simulink model "Full_system_6DOF"  (R2015b)
settings: Solver=ode3  StartTime=0.0  StopTime=30  FixedStep=0.001  RelTol=1e-3
values from neighbouring files (symbols this model uses):
  CoM = [0,0.00934172358962716,0.00356822089773090]'    [init_sim_3DOF.m]    (also in init_sim_4DOF.m = [0,0,0]'; init_sim_6DOF.m = [0,-0.01,0]')
  OS_damping_rot = 0    [init_sim_4DOF.m]    (also in init_sim_6DOF.m)
  OS_damping_trans = 0    [init_sim_4DOF.m]    (also in init_sim_6DOF.m)
  OS_Inertia = 1e-9*[13894080.33 -19869.26 46055.05 ... (first row only)    [init_sim_1DOF.m]    (also in init_sim_3DOF.m; init_sim_4DOF.m; init_sim_6DOF.m = 1e-9*[15414004.18 -17587.97 46447.37)
  OS_init_omega = 0    [init_sim_1DOF.m]    (also in init_sim_3DOF.m; init_sim_4DOF.m = [0 0 0]'; init_sim_6DOF.m = [0 0 0]')
  OS_init_vel = [0,0,0]'    [init_sim_3DOF.m]    (also in init_sim_4DOF.m; init_sim_6DOF.m)
  OS_rotation = 0    [init_sim_1DOF.m]    (also in init_sim_3DOF.m; init_sim_4DOF.m = [0 0 0]'; init_sim_6DOF.m = [0 0 0]')
  OS_xyz_des = (ea2dcm(SC_xyz(1,:)',72*pi/180)*OS_xyz_0')'    [init_sim_3DOF.m]    (also in init_sim_4DOF.m; init_sim_6DOF.m)
  rot_gain = 1e-8    (= 1e-08)    [init_sim_3DOF.m]    (also in init_sim_4DOF.m; init_sim_6DOF.m)
  SROA_Inertia = 1e7*eye(3)    [init_sim_3DOF.m]    (also in init_sim_4DOF.m)
  SROA_Mass = 100000    [init_sim_3DOF.m]    (also in init_sim_4DOF.m)
  trans_gain = 1e-7    (= 1e-07)    [init_sim_3DOF.m]    (also in init_sim_4DOF.m; init_sim_6DOF.m)
undefined symbols (not defined in the file or in its folder): EM_mu, EM_xyz, origin, OS_Mass, OS_mu_0, OS_xyz_0, Quat_A0
libraries: vrlib x3, simulink x3, my_ACS_library x1
settings Model: Creator=Frances  LastModifiedBy=user
settings DataIOCC: SaveFormat=Array
settings DebuggingCC: MaxConsecutiveZCsMsg=none  SolverPrmCheckMsg=warning
settings HardwareCC: ProdBitPerPointer=32  ProdLargestAtomicFloat=None  ProdIntDivRoundTo=Undefined  ProdEndianess=Unspecified  ProdWordSize=32  ProdHWDeviceType=32-bit Generic
settings GRTTargetCC: GeneratePreprocessorConditionals=Disable all
settings ConfigComp: CovModelRefEnable=Off  CovSFcnEnable=off

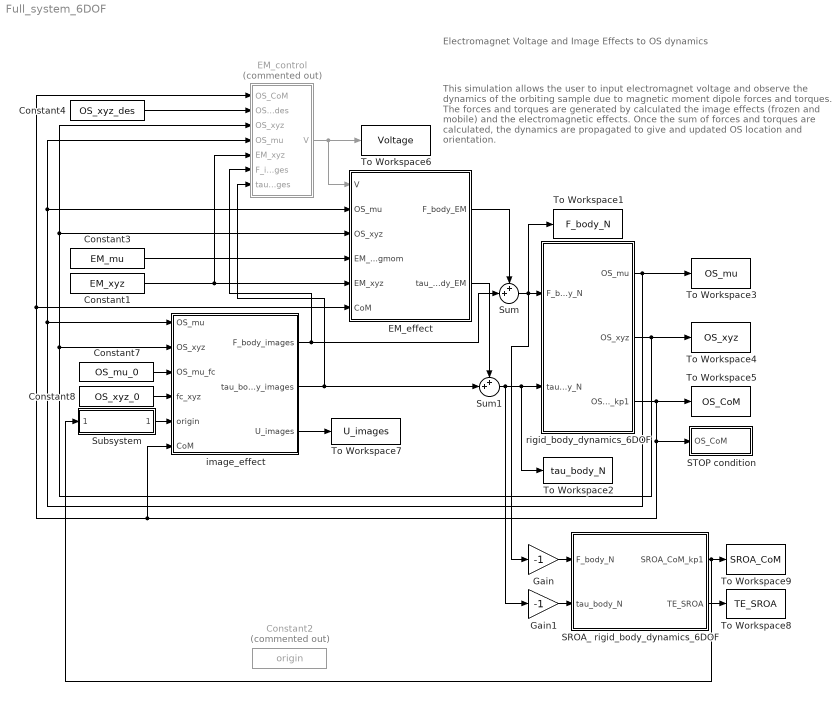
== system Full_system_6DOF ==
  note: This simulation allows the user to input electromagnet voltage and observe
      | the dynamics of the orbiting sample due to magnetic moment dipole forces
      | and torques. The forces and torques are generated by calculated the image
      | effects (frozen and mobile) and the electromagnetic effects. Once the sum
      | of forces and torques are calculated, the dynamics are propagated to give
      | and updated OS location and orientation.
  note: Electromagnet Voltage and Image Effects
      | to OS dynamics
  Constant1 : Constant  Value=EM_xyz
  Constant2 : Constant  Commented=on  Value=origin
  Constant3 : Constant  Value=EM_mu
  Constant4 : Constant  Value=OS_xyz_des
  Constant7 : Constant  Value=OS_mu_0  VectorParams1D=off
  Constant8 : Constant  Value=OS_xyz_0
  EM_control : Subsystem  Commented=on
  EM_effect : MATLAB Function  TreatAsAtomicUnit=on
  Gain : Gain  Gain=-1
  Gain1 : Gain  Gain=-1
  SROA_ rigid_body_dynamics_6DOF : Subsystem
  STOP condition : Subsystem
  Subsystem : Subsystem
  Sum : Sum  Inputs=++|
  Sum1 : Sum  Inputs=++|
  To Workspace1 : ToWorkspace  VariableName=F_body_N  SaveFormat=Timeseries  SampleTime=-1
  To Workspace2 : ToWorkspace  VariableName=tau_body_N  SaveFormat=Timeseries  SampleTime=-1
  To Workspace3 : ToWorkspace  VariableName=OS_mu  SaveFormat=Timeseries  SampleTime=-1
  To Workspace4 : ToWorkspace  VariableName=OS_xyz  SaveFormat=Timeseries  SampleTime=-1
  To Workspace5 : ToWorkspace  VariableName=OS_CoM  SaveFormat=Timeseries  SampleTime=-1
  To Workspace6 : ToWorkspace  VariableName=Voltage  SaveFormat=Timeseries  SampleTime=-1
  To Workspace7 : ToWorkspace  VariableName=U_images  SaveFormat=Timeseries  SampleTime=-1
      settings: Save2DSignal=2-D array (concatenate along first dimension)
  To Workspace8 : ToWorkspace  VariableName=TE_SROA  SaveFormat=Timeseries  SampleTime=-1
  To Workspace9 : ToWorkspace  VariableName=SROA_CoM  SaveFormat=Timeseries  SampleTime=-1
  image_effect : MATLAB Function  TreatAsAtomicUnit=on
  "rigid_body_dynamics_6DOF " : Subsystem
  wires:
  Constant3/1 -> EM_effect/4(EM_magmom)
  Constant1/1 -> EM_effect/5(EM_xyz), EM_control/5(EM_xyz)
  Subsystem/1(SROA_origin) -> image_effect/5(origin)
  Constant7/1 -> image_effect/3(OS_mu_fc)
  Constant8/1 -> image_effect/4(fc_xyz)
  image_effect/1(F_body_images) -> EM_control/6(F_images), Sum/2
  EM_effect/1(F_body_EM) -> Sum/1
  image_effect/2(tau_body_images) -> Sum1/2, EM_control/7(tau_images)
  EM_effect/2(tau_body_EM) -> Sum1/1
  Sum/1 -> To Workspace1/1, Gain/1, "rigid_body_dynamics_6DOF "/1(F_body_N)
  Sum1/1 -> Gain1/1, To Workspace2/1, "rigid_body_dynamics_6DOF "/2(tau_body_N)
  "rigid_body_dynamics_6DOF "/1(OS_mu) -> To Workspace3/1, EM_control/4(OS_mu), EM_effect/2(OS_mu), image_effect/1(OS_mu)
  "rigid_body_dynamics_6DOF "/2(OS_xyz) -> To Workspace4/1, EM_effect/3(OS_xyz), EM_control/3(OS_xyz), image_effect/2(OS_xyz)
  image_effect/3(U_images) -> To Workspace7/1
  "rigid_body_dynamics_6DOF "/3(OS_CoM_kp1) -> image_effect/6(CoM), EM_control/1(OS_CoM), EM_effect/6(CoM), STOP condition/1(OS_CoM), To Workspace5/1
  EM_control/1(V) -> EM_effect/1(V), To Workspace6/1
  Constant4/1 -> EM_control/2(OS_xyz_des)
  Gain/1 -> SROA_ rigid_body_dynamics_6DOF/1(F_body_N)
  Gain1/1 -> SROA_ rigid_body_dynamics_6DOF/2(tau_body_N)
  SROA_ rigid_body_dynamics_6DOF/2(TE_SROA) -> To Workspace8/1
  SROA_ rigid_body_dynamics_6DOF/1(SROA_CoM_kp1) -> Subsystem/1(SROA_CoM), To Workspace9/1

== system Full_system_6DOF/EM_control ==
  OS_CoM : Inport
  OS_xyz_des : Inport  Port=2
  OS_xyz : Inport  Port=3
  OS_mu : Inport  Port=4
  EM_xyz : Inport  Port=5
  F_images : Inport  Port=6
  tau_images : Inport  Port=7
  Display : Display
  calculate_V : Subsystem
  desired : Subsystem
  V : Outport
  wires:
  OS_xyz/1 -> desired/3(OS_xyz)
  OS_mu/1 -> desired/4(OS_mu)
  EM_xyz/1 -> desired/5(EM_xyz)
  OS_xyz_des/1 -> desired/2(OS_xyz_des)
  OS_CoM/1 -> desired/1(OS_CoM)
  calculate_V/1(V) -> Display/1, V/1
  F_images/1 -> desired/6(F_images)
  tau_images/1 -> desired/7(tau_images)
  desired/1(F_des) -> calculate_V/1(F_em)
  desired/2(tau_des) -> calculate_V/2(tau_em)
  desired/3(d/dV) -> calculate_V/3(dV)

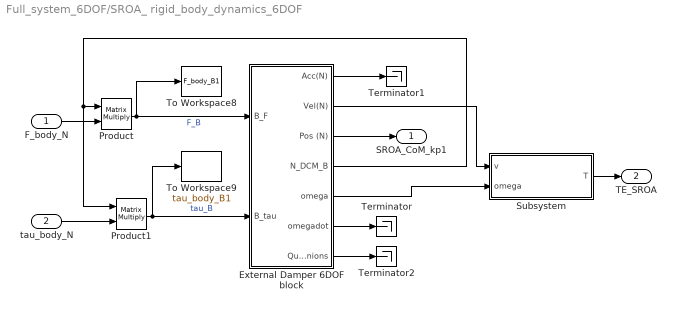
== system Full_system_6DOF/SROA_ rigid_body_dynamics_6DOF ==
  F_body_N : Inport
  tau_body_N : Inport  Port=2
  External Damper 6DOF block : Subsystem
  Product : Product  Multiplication=Matrix(*)
  Product1 : Product  Multiplication=Matrix(*)
  Subsystem : Subsystem
  Terminator : Terminator
  Terminator1 : Terminator
  Terminator2 : Terminator
  To Workspace8 : ToWorkspace  VariableName=F_body_B1  SaveFormat=Timeseries  SampleTime=-1
  To Workspace9 : ToWorkspace  VariableName=tau_body_B1  SaveFormat=Timeseries  SampleTime=-1
  SROA_CoM_kp1 : Outport
  TE_SROA : Outport  Port=2  PortDimensions=1
  wires:
  External Damper 6DOF block/1(Acc(N)) -> Terminator1/1
  External Damper 6DOF block/6(omegadot) -> Terminator/1
  tau_body_N/1 -> Product1/2
  F_body_N/1 -> Product/2
  External Damper 6DOF block/4(N_DCM_B) -> Product1/1, Product/1
  Product1/1 -> External Damper 6DOF block/2(B_tau), To Workspace9/1  "tau_B"
  Product/1 -> To Workspace8/1, External Damper 6DOF block/1(B_F)  "F_B"
  External Damper 6DOF block/3(Pos (N)) -> SROA_CoM_kp1/1
  Subsystem/1(T) -> TE_SROA/1
  External Damper 6DOF block/2(Vel(N)) -> Subsystem/1(v)
  External Damper 6DOF block/5(omega) -> Subsystem/2(omega)
  External Damper 6DOF block/7(Quaternions) -> Terminator2/1

== system Full_system_6DOF/STOP condition ==
  OS_CoM : Inport
  Compare To Constant : simulink/Logic and Bit Operations/Compare To Constant  relop=>  const=0.1  OutDataTypeStr=boolean
  Stop Simulation : Stop
  norm : Fcn  Expr=sqrt(u(1)^2+u(2)^2+u(3)^2)
  wires:
  Compare To Constant/1 -> Stop Simulation/1
  norm/1 -> Compare To Constant/1
  OS_CoM/1 -> norm/1

== system Full_system_6DOF/Subsystem ==
  SROA_CoM : Inport
  Constant2 : Constant  Value=origin
  MATLAB Function : MATLAB Function  TreatAsAtomicUnit=on
  SROA_origin : Outport
  wires:
  Constant2/1 -> MATLAB Function/1(origin)
  SROA_CoM/1 -> MATLAB Function/2(CoM)
  MATLAB Function/1(origin_new) -> SROA_origin/1

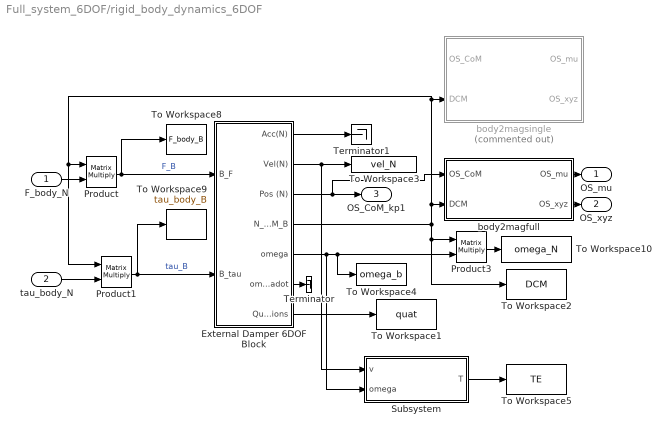
== system Full_system_6DOF/rigid_body_dynamics_6DOF  ==
  F_body_N : Inport
  tau_body_N : Inport  Port=2
  External Damper 6DOF Block : Subsystem
  Product : Product  Multiplication=Matrix(*)
  Product1 : Product  Multiplication=Matrix(*)
  Product3 : Product  Multiplication=Matrix(*)
  Subsystem : Subsystem
  Terminator : Terminator
  Terminator1 : Terminator
  To Workspace1 : ToWorkspace  VariableName=quat  SaveFormat=Timeseries  SampleTime=-1
  To Workspace10 : ToWorkspace  VariableName=omega_N  SaveFormat=Timeseries  SampleTime=-1
  To Workspace2 : ToWorkspace  VariableName=DCM  SaveFormat=Structure With Time  SampleTime=-1
  To Workspace3 : ToWorkspace  VariableName=vel_N  SaveFormat=Timeseries  SampleTime=-1
  To Workspace4 : ToWorkspace  VariableName=omega_b  SaveFormat=Timeseries  SampleTime=-1
  To Workspace5 : ToWorkspace  VariableName=TE  SaveFormat=Timeseries  SampleTime=-1
  To Workspace8 : ToWorkspace  VariableName=F_body_B  SaveFormat=Timeseries  SampleTime=-1
  To Workspace9 : ToWorkspace  VariableName=tau_body_B  SaveFormat=Timeseries  SampleTime=-1
  body2magfull : MATLAB Function  TreatAsAtomicUnit=on
  body2magsingle : MATLAB Function  Commented=on  TreatAsAtomicUnit=on
  OS_mu : Outport
  OS_xyz : Outport  Port=2
  OS_CoM_kp1 : Outport  Port=3
  wires:
  External Damper 6DOF Block/1(Acc(N)) -> Terminator1/1
  External Damper 6DOF Block/6(omegadot) -> Terminator/1
  External Damper 6DOF Block/2(Vel(N)) -> Subsystem/1(v), To Workspace3/1
  body2magfull/2(OS_xyz) -> OS_xyz/1
  body2magfull/1(OS_mu) -> OS_mu/1
  tau_body_N/1 -> Product1/2
  F_body_N/1 -> Product/2
  External Damper 6DOF Block/4(N_DCM_B) -> body2magfull/2(DCM), body2magsingle/2(DCM), Product1/1, Product/1, Product3/1, To Workspace2/1
  Product1/1 -> External Damper 6DOF Block/2(B_tau), To Workspace9/1  "tau_B"
  Product/1 -> External Damper 6DOF Block/1(B_F), To Workspace8/1  "F_B"
  External Damper 6DOF Block/3(Pos (N)) -> OS_CoM_kp1/1, body2magfull/1(OS_CoM)
  Product3/1 -> To Workspace10/1
  External Damper 6DOF Block/5(omega) -> Product3/2, To Workspace4/1, Subsystem/2(omega)
  External Damper 6DOF Block/7(Quaternions) -> To Workspace1/1
  Subsystem/1(T) -> To Workspace5/1

== system Full_system_6DOF/EM_control/calculate_V ==
  F_em : Inport
  tau_em : Inport  Port=2
  dV : Inport  Port=3
  Abs : Abs
  Divide : Product  Inputs=*/
  Gain : Gain  Gain=12
  MATLAB Function : MATLAB Function  TreatAsAtomicUnit=on
  MinMax : MinMax  Function=max
  Saturation : Saturate  Commented=on  UpperLimit=12  LowerLimit=-12  ZeroCross=off
  V : Outport
  wires:
  dV/1 -> MATLAB Function/3(dV)
  tau_em/1 -> MATLAB Function/2(tau_em)
  F_em/1 -> MATLAB Function/1(F_em)
  MinMax/1 -> Divide/2
  Abs/1 -> MinMax/1
  Divide/1 -> Gain/1
  MATLAB Function/1(V) -> Abs/1, Divide/1
  Gain/1 -> V/1

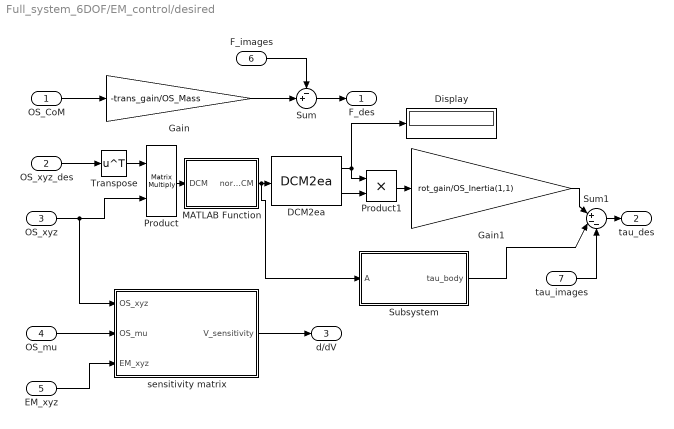
== system Full_system_6DOF/EM_control/desired ==
  OS_CoM : Inport
  OS_xyz_des : Inport  Port=2
  OS_xyz : Inport  Port=3
  OS_mu : Inport  Port=4
  EM_xyz : Inport  Port=5
  F_images : Inport  Port=6
  tau_images : Inport  Port=7
  DCM2ea : my_ACS_library/attitude conversions/DCM2ea
  Display : Display
  Gain : Gain  Gain=-trans_gain/OS_Mass
  Gain1 : Gain  Gain=rot_gain/OS_Inertia(1,1)
  MATLAB Function : MATLAB Function  TreatAsAtomicUnit=on
  Product : Product  Multiplication=Matrix(*)
  Product1 : Product
  Subsystem : Subsystem
  Sum : Sum  Inputs=-+|
  Sum1 : Sum  Inputs=|+--
  Transpose : Math  Operator=transpose  SaturateOnIntegerOverflow=on
  sensitivity matrix : MATLAB Function  TreatAsAtomicUnit=on
  F_des : Outport
  tau_des : Outport  Port=2
  d/dV : Outport  Port=3
  wires:
  sensitivity matrix/1(V_sensitivity) -> d/dV/1
  OS_xyz_des/1 -> Transpose/1
  Transpose/1 -> Product/1
  OS_CoM/1 -> Gain/1
  EM_xyz/1 -> sensitivity matrix/3(EM_xyz)
  OS_xyz/1 -> Product/2, sensitivity matrix/1(OS_xyz)
  OS_mu/1 -> sensitivity matrix/2(OS_mu)
  Product/1 -> MATLAB Function/1(DCM)
  MATLAB Function/1(normDCM) -> Subsystem/1(A), DCM2ea/1
  Product1/1 -> Gain1/1
  DCM2ea/1 -> Product1/1, Display/1
  DCM2ea/2 -> Product1/2
  Gain/1 -> Sum/2
  Sum/1 -> F_des/1
  F_images/1 -> Sum/1
  Sum1/1 -> tau_des/1
  Gain1/1 -> Sum1/1
  tau_images/1 -> Sum1/3
  Subsystem/1(tau_body) -> Sum1/2

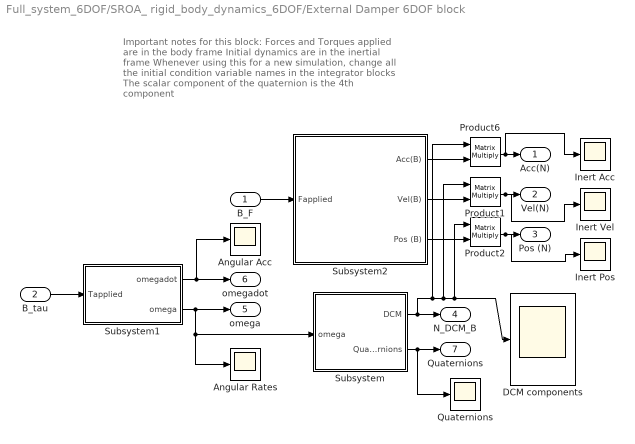
== system Full_system_6DOF/SROA_ rigid_body_dynamics_6DOF/External Damper 6DOF block ==
  note: Important notes for this block:
      | Forces and Torques applied are in the body frame
      | Initial dynamics are in the inertial frame
      | Whenever using this for a new simulation, change all the initial condition variable names in the integrator blocks
      | The scalar component of the quaternion is the 4th component
  B_F : Inport
  B_tau : Inport  Port=2
  Angular Acc : Scope
  Angular Rates : Scope
  DCM components : Scope
  Inert Acc : Scope
  Inert Pos : Scope
  Inert Vel : Scope
  Product1 : Product  Multiplication=Matrix(*)  RndMeth=Zero
  Product2 : Product  Multiplication=Matrix(*)  RndMeth=Zero
  Product6 : Product  Multiplication=Matrix(*)  RndMeth=Zero
  "Quaternions " : Scope
  Subsystem : Subsystem
  Subsystem1 : Subsystem
  Subsystem2 : Subsystem
  Acc(N) : Outport
  Vel(N) : Outport  Port=2
  Pos (N) : Outport  Port=3
  N_DCM_B : Outport  Port=4
  omega : Outport  Port=5
  omegadot : Outport  Port=6
  Quaternions : Outport  Port=7
  wires:
  Subsystem/2(Quaternions) -> Quaternions/1, "Quaternions "/1
  Subsystem/1(DCM) -> N_DCM_B/1, Product6/1, Product1/1, Product2/1, DCM components/1
  Subsystem1/1(omegadot) -> omegadot/1, Angular Acc/1
  Subsystem1/2(omega) -> Angular Rates/1, Subsystem/1(omega), omega/1
  B_F/1 -> Subsystem2/1(Fapplied)
  B_tau/1 -> Subsystem1/1(Tapplied)
  Product6/1 -> Inert Acc/1, Acc(N)/1
  Product1/1 -> Inert Vel/1, Vel(N)/1
  Product2/1 -> Inert Pos/1, Pos (N)/1
  Subsystem2/2(Vel(B)) -> Product1/2
  Subsystem2/1(Acc(B)) -> Product6/2
  Subsystem2/3(Pos (B)) -> Product2/2

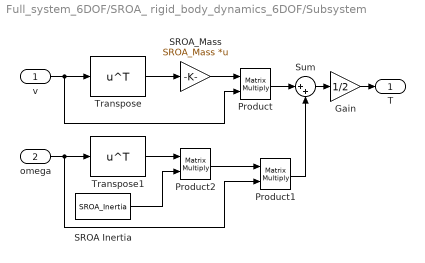
== system Full_system_6DOF/SROA_ rigid_body_dynamics_6DOF/Subsystem ==
  v : Inport
  omega : Inport  Port=2
  Gain : Gain  Gain=1/2
  Product : Product  Multiplication=Matrix(*)
  Product1 : Product  Multiplication=Matrix(*)
  Product2 : Product  Multiplication=Matrix(*)
  SROA Inertia : Constant  Value=SROA_Inertia
  SROA_Mass : Gain  Gain=SROA_Mass  Multiplication=Matrix(K*u)
  Sum : Sum  Inputs=|++
  Transpose : Math  Operator=transpose  SaturateOnIntegerOverflow=on
  Transpose1 : Math  Operator=transpose  SaturateOnIntegerOverflow=on
  T : Outport
  wires:
  v/1 -> Product/2, Transpose/1
  Transpose/1 -> SROA_Mass/1
  SROA_Mass/1 -> Product/1
  Sum/1 -> Gain/1
  Gain/1 -> T/1
  omega/1 -> Product1/2, Transpose1/1
  Transpose1/1 -> Product2/1
  Product2/1 -> Product1/1
  Product/1 -> Sum/1
  Product1/1 -> Sum/2
  SROA Inertia/1 -> Product2/2

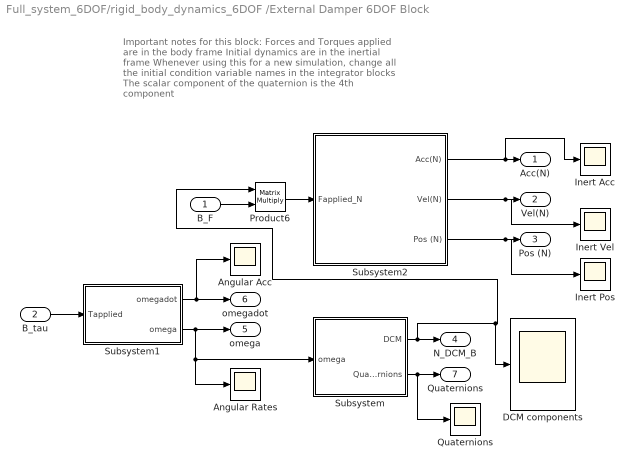
== system Full_system_6DOF/rigid_body_dynamics_6DOF /External Damper 6DOF Block ==
  note: Important notes for this block:
      | Forces and Torques applied are in the body frame
      | Initial dynamics are in the inertial frame
      | Whenever using this for a new simulation, change all the initial condition variable names in the integrator blocks
      | The scalar component of the quaternion is the 4th component
  B_F : Inport
  B_tau : Inport  Port=2
  Angular Acc : Scope
  Angular Rates : Scope
  DCM components : Scope
  Inert Acc : Scope
  Inert Pos : Scope
  Inert Vel : Scope
  Product6 : Product  Multiplication=Matrix(*)  RndMeth=Zero
  "Quaternions " : Scope
  Subsystem : Subsystem
  Subsystem1 : Subsystem
  Subsystem2 : Subsystem
  Acc(N) : Outport
  Vel(N) : Outport  Port=2  PortDimensions=[3 1]
  Pos (N) : Outport  Port=3
  N_DCM_B : Outport  Port=4
  omega : Outport  Port=5  PortDimensions=[3 1]
  omegadot : Outport  Port=6
  Quaternions : Outport  Port=7
  wires:
  Product6/1 -> Subsystem2/1(Fapplied_N)
  Subsystem/2(Quaternions) -> Quaternions/1, "Quaternions "/1
  Subsystem/1(DCM) -> N_DCM_B/1, Product6/1, DCM components/1
  Subsystem1/1(omegadot) -> omegadot/1, Angular Acc/1
  Subsystem1/2(omega) -> Angular Rates/1, Subsystem/1(omega), omega/1
  B_tau/1 -> Subsystem1/1(Tapplied)
  Subsystem2/1(Acc(N)) -> Inert Acc/1, Acc(N)/1
  Subsystem2/2(Vel(N)) -> Inert Vel/1, Vel(N)/1
  Subsystem2/3(Pos (N)) -> Inert Pos/1, Pos (N)/1
  B_F/1 -> Product6/2

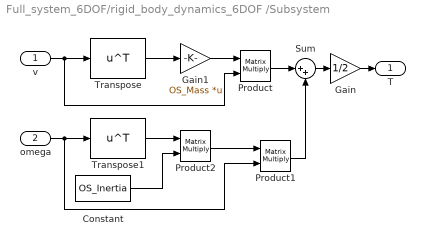
== system Full_system_6DOF/rigid_body_dynamics_6DOF /Subsystem ==
  v : Inport
  omega : Inport  Port=2
  Constant : Constant  Value=OS_Inertia
  Gain : Gain  Gain=1/2
  Gain1 : Gain  Gain=OS_Mass  Multiplication=Matrix(K*u)
  Product : Product  Multiplication=Matrix(*)
  Product1 : Product  Multiplication=Matrix(*)
  Product2 : Product  Multiplication=Matrix(*)
  Sum : Sum  Inputs=|++
  Transpose : Math  Operator=transpose  SaturateOnIntegerOverflow=on
  Transpose1 : Math  Operator=transpose  SaturateOnIntegerOverflow=on
  T : Outport  PortDimensions=1
  wires:
  v/1 -> Product/2, Transpose/1
  Transpose/1 -> Gain1/1
  Gain1/1 -> Product/1
  Sum/1 -> Gain/1
  Gain/1 -> T/1
  omega/1 -> Product1/2, Transpose1/1
  Transpose1/1 -> Product2/1
  Product2/1 -> Product1/1
  Product/1 -> Sum/1
  Product1/1 -> Sum/2
  Constant/1 -> Product2/2

== system Full_system_6DOF/EM_control/desired/Subsystem ==
  A : Inport
  Constant : Constant  Value=OS_Inertia
  Cross Product : vrlib/Utilities/Cross Product
  Derivative : Derivative
  Display : Display
  MATLAB Function1 : MATLAB Function  TreatAsAtomicUnit=on
  Product : Product  Multiplication=Matrix(*)
  tau_body : Outport
  wires:
  Derivative/1 -> MATLAB Function1/2(dA)
  A/1 -> Derivative/1, MATLAB Function1/1(A)
  MATLAB Function1/1(omega) -> Product/2, Display/1, Cross Product/1
  Product/1 -> Cross Product/2
  Cross Product/1 -> tau_body/1
  Constant/1 -> Product/1

== system Full_system_6DOF/SROA_ rigid_body_dynamics_6DOF/External Damper 6DOF block/Subsystem ==
  omega : Inport
  Divide : Product  Inputs=*/
  Initialize quaternion : Subsystem
  Integrator1 : Integrator  InitialConditionSource=external  InitialCondition=Quat_A0
  Quat Norm : Scope
  STOP condition : Subsystem
  find the derivative of the quaternion : MATLAB Function  TreatAsAtomicUnit=on
  norm : Fcn  Expr=u(1)^2+u(2)^2+u(3)^2+u(4)^2
  quat2DCM : MATLAB Function  TreatAsAtomicUnit=on
  DCM : Outport
  Quaternions : Outport  Port=2
  wires:
  Initialize quaternion/1(qinit) -> Integrator1/2
  quat2DCM/1(DCM) -> DCM/1
  find the derivative of the quaternion/1(qdot) -> STOP condition/1(qdot), Integrator1/1
  Divide/1 -> quat2DCM/1(q), find the derivative of the quaternion/2(q), Quat Norm/1, Quaternions/1
  omega/1 -> find the derivative of the quaternion/1(w)
  Integrator1/1 -> Divide/1, norm/1
  norm/1 -> Divide/2

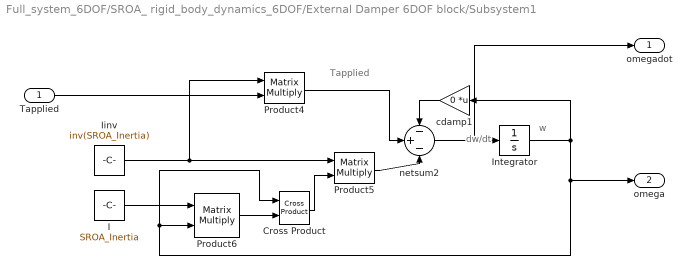
== system Full_system_6DOF/SROA_ rigid_body_dynamics_6DOF/External Damper 6DOF block/Subsystem1 ==
  note: dw/dt
  note: w
  note: Tapplied
  Tapplied : Inport
  Cross Product : vrlib/Utilities/Cross Product
  I : Constant  Value=SROA_Inertia  VectorParams1D=off
  Iinv : Constant  Value=inv(SROA_Inertia)  VectorParams1D=off
  Integrator : Integrator  InitialCondition=[0 0 0]'
  Product4 : Product  Multiplication=Matrix(*)  RndMeth=Zero
  Product5 : Product  Multiplication=Matrix(*)  RndMeth=Zero
  Product6 : Product  Multiplication=Matrix(*)  RndMeth=Zero
  cdamp1 : Gain  Gain=0  Multiplication=Matrix(K*u)
  netsum2 : Sum  Inputs=-+-  SaturateOnIntegerOverflow=on  InputSameDT=on  OutDataTypeStr=Inherit: Same as first input
  omegadot : Outport
  omega : Outport  Port=2
  wires:
  Cross Product/1 -> Product5/2
  cdamp1/1 -> netsum2/1
  Product4/1 -> netsum2/2
  Product5/1 -> netsum2/3
  Iinv/1 -> Product4/1, Product5/1
  Tapplied/1 -> Product4/2
  Product6/1 -> Cross Product/2
  I/1 -> Product6/1
  netsum2/1 -> Integrator/1, omegadot/1
  Integrator/1 -> omega/1, Cross Product/1, Product6/2, cdamp1/1

== system Full_system_6DOF/SROA_ rigid_body_dynamics_6DOF/External Damper 6DOF block/Subsystem2 ==
  note: dVb/dt
  note: Vb
  note: Fapplied
  Fapplied : Inport
  Integrator1 : Integrator  InitialCondition=[0 0 0]'
  Integrator2 : Integrator  InitialCondition=[0 0 0]'
  Mass_A0 inv : Gain  Gain=1/SROA_Mass  Multiplication=Matrix(K*u)
  Sum : Sum  Inputs=-+|  SaturateOnIntegerOverflow=on
  cdamp : Gain  Gain=OS_damping_trans  Multiplication=Matrix(K*u)
  Acc(B) : Outport
  Vel(B) : Outport  Port=2
  Pos (B) : Outport  Port=3
  wires:
  cdamp/1 -> Sum/1
  Mass_A0 inv/1 -> Sum/2
  Fapplied/1 -> Mass_A0 inv/1
  Sum/1 -> Integrator1/1, Acc(B)/1
  Integrator2/1 -> Pos (B)/1
  Integrator1/1 -> cdamp/1, Integrator2/1, Vel(B)/1

== system Full_system_6DOF/rigid_body_dynamics_6DOF /External Damper 6DOF Block/Subsystem ==
  omega : Inport
  Divide : Product  Inputs=*/
  Initialize quaternion : Subsystem
  Integrator3 : Integrator  InitialConditionSource=external  InitialCondition=Quat_A0
  Quat Norm : Scope
  STOP condition : Subsystem
  find the derivative of the quaternion : MATLAB Function  TreatAsAtomicUnit=on
  norm : Fcn  Expr=u(1)^2+u(2)^2+u(3)^2+u(4)^2
  quat2DCM : MATLAB Function  TreatAsAtomicUnit=on
  DCM : Outport
  Quaternions : Outport  Port=2
  wires:
  Initialize quaternion/1(qinit) -> Integrator3/2
  quat2DCM/1(DCM) -> DCM/1
  find the derivative of the quaternion/1(qdot) -> STOP condition/1(qdot), Integrator3/1
  Divide/1 -> quat2DCM/1(q), Quaternions/1, find the derivative of the quaternion/2(q), Quat Norm/1
  Integrator3/1 -> Divide/1, norm/1
  omega/1 -> find the derivative of the quaternion/1(w)
  norm/1 -> Divide/2

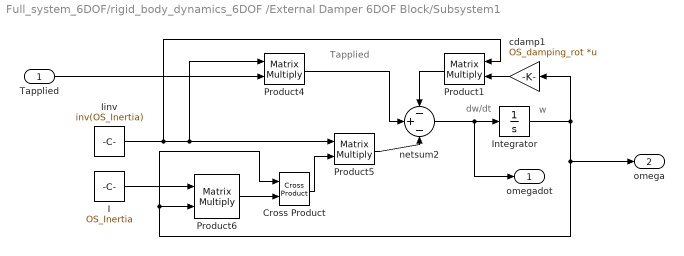
== system Full_system_6DOF/rigid_body_dynamics_6DOF /External Damper 6DOF Block/Subsystem1 ==
  note: dw/dt
  note: w
  note: Tapplied
  Tapplied : Inport
  Cross Product : vrlib/Utilities/Cross Product
  I : Constant  Value=OS_Inertia  VectorParams1D=off
  Iinv : Constant  Value=inv(OS_Inertia)  VectorParams1D=off
  Integrator : Integrator  InitialCondition=OS_init_omega
  Product{1,4..6} (4 alike) : Product  Multiplication=Matrix(*)  RndMeth=Zero
  cdamp1 : Gain  Gain=OS_damping_rot  Multiplication=Matrix(K*u)
  netsum2 : Sum  Inputs=-+-  SaturateOnIntegerOverflow=on  InputSameDT=on  OutDataTypeStr=Inherit: Same as first input
  omegadot : Outport
  omega : Outport  Port=2
  wires:
  Cross Product/1 -> Product5/2
  Product4/1 -> netsum2/2
  Product5/1 -> netsum2/3
  Iinv/1 -> Product1/1, Product4/1, Product5/1
  Tapplied/1 -> Product4/2
  Product6/1 -> Cross Product/2
  I/1 -> Product6/1
  netsum2/1 -> Integrator/1, omegadot/1
  Integrator/1 -> omega/1, Cross Product/1, Product6/2, cdamp1/1
  cdamp1/1 -> Product1/2
  Product1/1 -> netsum2/1

== system Full_system_6DOF/rigid_body_dynamics_6DOF /External Damper 6DOF Block/Subsystem2 ==
  note: dVn/dt
  note: Fapplied
  Fapplied_N : Inport
  Bounce : Subsystem
  Mass_A0 inv : Gain  Gain=1/OS_Mass  Multiplication=Matrix(K*u)
  Sum : Sum  Inputs=+-+|  SaturateOnIntegerOverflow=on
  To Workspace3 : ToWorkspace  VariableName=bounce_force  SaveFormat=Timeseries  SampleTime=-1
  cdamp : Gain  Gain=OS_damping_trans  Multiplication=Matrix(K*u)
  double integral : Subsystem
  Acc(N) : Outport
  Vel(N) : Outport  Port=2
  Pos (N) : Outport  Port=3
  wires:
  double integral/2(Velocity) -> Vel(N)/1, cdamp/1
  double integral/1(Position) -> Bounce/1(OS_CoM), Pos (N)/1
  Mass_A0 inv/1 -> double integral/1(Acceleration), Acc(N)/1
  Sum/1 -> Mass_A0 inv/1
  Bounce/1(Force) -> To Workspace3/1, Sum/1
  Fapplied_N/1 -> Sum/3
  cdamp/1 -> Sum/2

== system Full_system_6DOF/SROA_ rigid_body_dynamics_6DOF/External Damper 6DOF block/Subsystem/Initialize quaternion ==
  Initial Euler Angles : Constant  Value=OS_rotation
  Selector1 : Selector  InputPortWidth=3  IndexOptions=Index vector (dialog)  Indices=[3 2 1]  OutputSizes=1
  yaw,pitch,roll to quat : MATLAB Function  TreatAsAtomicUnit=on
  qinit : Outport
  wires:
  yaw,pitch,roll to quat/1(q) -> qinit/1
  Selector1/1 -> yaw,pitch,roll to quat/1(angles)
  Initial Euler Angles/1 -> Selector1/1

== system Full_system_6DOF/SROA_ rigid_body_dynamics_6DOF/External Damper 6DOF block/Subsystem/STOP condition ==
  qdot : Inport
  Compare To Constant : simulink/Logic and Bit Operations/Compare To Constant  relop=>  const=10  OutDataTypeStr=boolean
  Stop Simulation : Stop
  norm : Fcn  Expr=sqrt(u(1)^2+u(2)^2+u(3)^2)
  wires:
  Compare To Constant/1 -> Stop Simulation/1
  norm/1 -> Compare To Constant/1
  qdot/1 -> norm/1

== system Full_system_6DOF/rigid_body_dynamics_6DOF /External Damper 6DOF Block/Subsystem/Initialize quaternion ==
  Initial Euler Angles : Constant  Value=OS_rotation
  Selector1 : Selector  InputPortWidth=3  IndexOptions=Index vector (dialog)  Indices=[3 2 1]  OutputSizes=1
  yaw,pitch,roll to quat : MATLAB Function  TreatAsAtomicUnit=on
  qinit : Outport
  wires:
  yaw,pitch,roll to quat/1(q) -> qinit/1
  Selector1/1 -> yaw,pitch,roll to quat/1(angles)
  Initial Euler Angles/1 -> Selector1/1

== system Full_system_6DOF/rigid_body_dynamics_6DOF /External Damper 6DOF Block/Subsystem/STOP condition ==
  qdot : Inport
  Compare To Constant : simulink/Logic and Bit Operations/Compare To Constant  relop=>  const=10  OutDataTypeStr=boolean
  Stop Simulation : Stop
  norm : Fcn  Expr=sqrt(u(1)^2+u(2)^2+u(3)^2)
  wires:
  Compare To Constant/1 -> Stop Simulation/1
  norm/1 -> Compare To Constant/1
  qdot/1 -> norm/1

== system Full_system_6DOF/rigid_body_dynamics_6DOF /External Damper 6DOF Block/Subsystem2/Bounce ==
  OS_CoM : Inport
  cone : Subsystem  Commented=on
  pocket : Subsystem
  Force : Outport
  wires:
  OS_CoM/1 -> pocket/1(OS_CoM)
  pocket/1(Force) -> Force/1

== system Full_system_6DOF/rigid_body_dynamics_6DOF /External Damper 6DOF Block/Subsystem2/double integral ==
  note: if you want the bounce, extract it from an older sim version 6/22/2015
  Acceleration : Inport
  Integrator1 : Integrator  InitialCondition=CoM
  Integrator2 : Integrator  InitialCondition=OS_init_vel  UpperSaturationLimit=100  LowerSaturationLimit=-100
  Pos : Scope
  pos : ToWorkspace  VariableName=pos  SaveFormat=Timeseries  SampleTime=-1
  Position : Outport
  Velocity : Outport  Port=2
  wires:
  Acceleration/1 -> Integrator2/1
  Integrator2/1 -> Integrator1/1, Velocity/1  "Velocity"
  Integrator1/1 -> pos/1, Position/1, Pos/1  "Position"

== system Full_system_6DOF/rigid_body_dynamics_6DOF /External Damper 6DOF Block/Subsystem2/Bounce/cone ==
  OS_CoM : Inport
  Gain : Gain  Gain=-2
  Product : Product
  Subsystem : Subsystem
  pos to norm vec : Subsystem
  Force : Outport
  wires:
  Gain/1 -> Force/1
  Subsystem/1(k(x)) -> Product/1
  Product/1 -> Gain/1
  OS_CoM/1 -> pos to norm vec/1(OS_CoM), Subsystem/1(OS_CoM)
  pos to norm vec/1(a_hat) -> Product/2

== system Full_system_6DOF/rigid_body_dynamics_6DOF /External Damper 6DOF Block/Subsystem2/Bounce/pocket ==
  OS_CoM : Inport
  Gain : Gain  Gain=-1
  Product : Product
  Subsystem : Subsystem
  Force : Outport
  wires:
  Gain/1 -> Force/1
  Subsystem/1(k(x)) -> Product/1
  Product/1 -> Gain/1
  OS_CoM/1 -> Subsystem/1(OS_CoM), Product/2

== system Full_system_6DOF/rigid_body_dynamics_6DOF /External Damper 6DOF Block/Subsystem2/Bounce/cone/Subsystem ==
  OS_CoM : Inport
  Display : Display
  Fcn : Fcn  Expr=10*exp(10000*u)
  Subsystem : Subsystem
  k(x) : Outport
  wires:
  Fcn/1 -> k(x)/1
  Subsystem/1(x) -> Fcn/1, Display/1
  OS_CoM/1 -> Subsystem/1(OS_CoM)

== system Full_system_6DOF/rigid_body_dynamics_6DOF /External Damper 6DOF Block/Subsystem2/Bounce/cone/pos to norm vec ==
  OS_CoM : Inport
  Constant : Constant  Value=0.02
  Demux : Demux  Outputs=3
  Divide : Product  Inputs=*/
  Gain : Gain  Gain=2
  Gain1 : Gain  Gain=2
  Gain2 : Gain  Gain=2
  Mux : Mux  Inputs=3
  Sum : Sum  Inputs=|+-
  norm3x1 : Fcn  Expr=sqrt(u(1)^2+u(2)^2+u(3)^2)
  a_hat : Outport
  wires:
  OS_CoM/1 -> Demux/1
  Demux/1 -> Gain/1
  Gain2/1 -> Mux/3
  Demux/3 -> Gain2/1
  Demux/2 -> Gain1/1
  Gain/1 -> Mux/1
  Gain1/1 -> Sum/1
  Sum/1 -> Mux/2
  Constant/1 -> Sum/2
  Divide/1 -> a_hat/1
  Mux/1 -> norm3x1/1, Divide/1
  norm3x1/1 -> Divide/2

== system Full_system_6DOF/rigid_body_dynamics_6DOF /External Damper 6DOF Block/Subsystem2/Bounce/pocket/Subsystem ==
  OS_CoM : Inport
  Display : Display
  Fcn : Fcn  Expr=10*exp(10000*u)
  Subsystem : Subsystem
  k(x) : Outport
  wires:
  Fcn/1 -> k(x)/1
  Subsystem/1(x) -> Fcn/1, Display/1
  OS_CoM/1 -> Subsystem/1(OS_CoM)

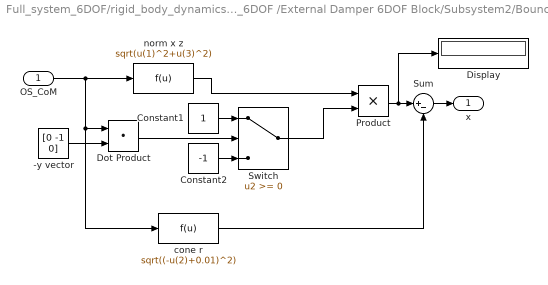
== system Full_system_6DOF/rigid_body_dynamics_6DOF /External Damper 6DOF Block/Subsystem2/Bounce/cone/Subsystem/Subsystem ==
  OS_CoM : Inport
  -y vector : Constant  Value=[0 -1 0]
  Constant1 : Constant
  Constant2 : Constant  Value=-1
  Display : Display
  Dot Product : DotProduct  InputSameDT=on  OutDataTypeStr=Inherit: Inherit via internal rule
  Product : Product
  Sum : Sum  Inputs=|+-
  Switch : Switch
  cone r : Fcn  Expr=sqrt((-u(2)+0.01)^2)
  norm x z : Fcn  Expr=sqrt(u(1)^2+u(3)^2)
  x : Outport
  wires:
  Switch/1 -> Product/2
  Constant2/1 -> Switch/3
  Constant1/1 -> Switch/1
  Product/1 -> Sum/1, Display/1
  Sum/1 -> x/1
  Dot Product/1 -> Switch/2
  OS_CoM/1 -> cone r/1, Dot Product/1, norm x z/1
  norm x z/1 -> Product/1
  -y vector/1 -> Dot Product/2
  cone r/1 -> Sum/2

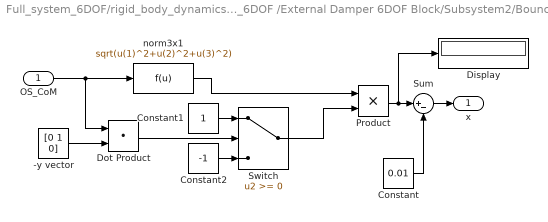
== system Full_system_6DOF/rigid_body_dynamics_6DOF /External Damper 6DOF Block/Subsystem2/Bounce/pocket/Subsystem/Subsystem ==
  OS_CoM : Inport
  -y vector : Constant  Value=[0 1 0]
  Constant : Constant  Value=0.01
  Constant1 : Constant
  Constant2 : Constant  Value=-1
  Display : Display
  Dot Product : DotProduct  InputSameDT=on  OutDataTypeStr=Inherit: Inherit via internal rule
  Product : Product
  Sum : Sum  Inputs=|+-
  Switch : Switch
  norm3x1 : Fcn  Expr=sqrt(u(1)^2+u(2)^2+u(3)^2)
  x : Outport
  wires:
  Switch/1 -> Product/2
  Constant2/1 -> Switch/3
  Constant1/1 -> Switch/1
  Product/1 -> Sum/1, Display/1
  Sum/1 -> x/1
  Constant/1 -> Sum/2
  Dot Product/1 -> Switch/2
  OS_CoM/1 -> Dot Product/1, norm3x1/1
  norm3x1/1 -> Product/1
  -y vector/1 -> Dot Product/2

== matlab function Full_system_6DOF/EM_control/calculate_V/MATLAB Function ==
  data: F_em input; V output; tau_em input; dV input
function V = voltage(F_em,tau_em,dV)
%#codegen

V=dV\[F_em;tau_em];
end

== matlab function Full_system_6DOF/EM_control/desired/sensitivity matrix ==
  data: OS_xyz input; V_sensitivity output; OS_mu input; EM_xyz input
function V_sensitivity=calculate_voltage(OS_xyz, OS_mu, EM_xyz)
%% Calculate the needed electromagnet voltage with a pseudoinverse
    %initialize a placeholder for the pseudoinverse
    V_sensitivity=zeros(6,6);
    
    %sift through all the electromagnets to back out portion of force
    %and torque generated from each individually
    for i=1:6 
        %initialize sum of electromagnet contribution acting on each
        %permanent magnet due to electromagnet i
        dF_tot=zeros(1,3); 
        dtau_tot=zeros(1,3);
        %calculate electromagnet affect on force and torque on body through
        %all the permanent magnets
        for j=1:size(OS_xyz,2) 
            %in this case, the magnetic moment dipole being acted on is the 
            %permanent magnet, following Villani convention
            mu_mag_i=OS_mu(j,:);
            pos_mag_i=OS_xyz(j,:);
            %the magnetic moment dipole acting on magnet i is the
            %electromagnet
            pos_mag_j=EM_xyz(i,:);
            mu_mag_j=-EM_xyz(i,:)/norm(EM_xyz(i,:));
            %calculate_dV is a variation of villani. Villani requires mu
            %components and the position vector between them. Within
            %calculate_dV, the electromagnet's magnetic dipole/voltage is
            %substituted for force and torque per unit Volt
            [dF_dV,dtau_dV]=calculate_dV(mu_mag_i,pos_mag_i,mu_mag_j,pos_mag_j);
            %sum over each permanent magnet
            dF_tot=dF_tot+dF_dV;
            dtau_tot=dtau_tot+dtau_dV+cross(dF_tot,pos_mag_i);
        end
        %fill in the portion of the pseudoinverse needed to calculate
        %electromagnetic contribution
        V_sensitivity(:,i)=[dF_tot';dtau_tot'];
    end
end

== matlab function Full_system_6DOF/rigid_body_dynamics_6DOF /body2magfull ==
  data: OS_CoM input; OS_mu output; DCM input; OS_xyz output
function [OS_mu,OS_xyz] = body2mag(OS_CoM,DCM)
%#codegen
tau=(1+sqrt(5))/2;
OS_xyz=[0 1 tau;
    -1 tau 0;
    1 tau 0;
    0 1 -tau;
    0 -1 tau;
    0 -1 -tau;
    1 -tau 0;
    -1 -tau 0;
    tau 0 1;
    tau 0 -1;
    -tau 0 -1;
    -tau 0 1];
%^the coordinate points of an icosahedron
D=20.3/100; %m the diameter of the OS
magd=1.905/100; %m the diameter of the 0.75 inch spherical magnets to use
rM=(D-magd)/2; %m this radius corresponds to the center of the magnets 
%so that the magnets are flush against the OS surface
OS_magmom=zeros(size(OS_xyz));
for i=1:size(OS_xyz,1)
    OS_magmom(i,:)=(DCM*OS_xyz(i,:)'/norm(OS_xyz(i,:)))';
    OS_xyz(i,:)=OS_magmom(i,:)*rM+OS_CoM';
end
%the permeability of free space, mu_0
mu_0=4*pi*10^-7; %N/A^2

%surface strength of the magnetic field of the dipole measured along its
%dipole axis taken from manufacturer's website
B_m=8815e-4; %Tesla

%distance from the center of the magnet to its surface
d_m=1.905/2/100; %m

%the estimated magnetic dipole moment magnitude for each magnet on the OS
%surface
OS_mu=2*pi*B_m*d_m^3/mu_0*OS_magmom;

== matlab function Full_system_6DOF/rigid_body_dynamics_6DOF /body2magsingle ==
  data: OS_CoM input; OS_mu output; DCM input; OS_xyz output
function [OS_mu,OS_xyz] = body2mag(OS_CoM,DCM)
%#codegen

OS_xyz=[0 0 0];

OS_magmom=zeros(size(OS_xyz));
for i=1:size(OS_xyz,1)
    OS_magmom(i,:)=(DCM*[0 0 -1]')';
    OS_xyz(i,:)=OS_CoM';
end

%xyz at this line corresponds to the coordinate points of the center of the
%small spherical magnets

%the permeability of free space, mu_0
mu_0=4*pi*10^-7; %N/A^2

%surface strength of the magnetic field of the dipole measured along its
%dipole axis taken from manufacturer's website
B_m=8815e-4; %Tesla

%distance from the center of the magnet to its surface
d_m=1.905/2/100; %m

%the estimated magnetic dipole moment magnitude for each magnet on the OS
%surface
OS_mu=2*pi*B_m*d_m^3/mu_0*OS_magmom;

== matlab function Full_system_6DOF/EM_control/desired/MATLAB Function ==
  data: DCM input; normDCM output
function normDCM = normA(DCM)
%#codegen
normDCM=[DCM(:,1)/norm(DCM(:,1)) DCM(:,2)/norm(DCM(:,2)) DCM(:,3)/norm(DCM(:,3))];

== matlab function Full_system_6DOF/EM_control/desired/Subsystem/MATLAB Function1 ==
  data: A input; omega output; dA input
function omega = DCM2omega(A,dA)
%#codegen
W=dA/A;
omega=[W(3,2) W(1,3) W(2,1)]';

== matlab function Full_system_6DOF/Subsystem/MATLAB Function ==
  data: origin input; origin_new output; CoM input
function origin_new = fcn(origin,CoM)
%#codegen
origin_new=zeros(3,3);
for i=1:3
    origin_new(i,:)=origin(i,:)+CoM';
end

== matlab function Full_system_6DOF/SROA_ rigid_body_dynamics_6DOF/External Damper 6DOF block/Subsystem/Initialize quaternion/yaw,pitch,roll to quat ==
  data: q output; angles input
function q = ang2quat(angles)
%#eml
phi=angles(1);
theta=angles(2);
psi=angles(3);
q1=sin(phi/2)*cos(theta/2)*cos(psi/2)-cos(phi/2)*sin(theta/2)*sin(psi/2);
q2=cos(phi/2)*sin(theta/2)*cos(psi/2)+sin(phi/2)*cos(theta/2)*sin(psi/2);
q3=cos(phi/2)*cos(theta/2)*sin(psi/2)-sin(phi/2)*cos(theta/2)*sin(psi/2);
q4=cos(phi/2)*cos(theta/2)*cos(psi/2)+sin(phi/2)*sin(theta/2)*sin(psi/2);
q=[q1 q2 q3 q4]';

== matlab function Full_system_6DOF/SROA_ rigid_body_dynamics_6DOF/External Damper 6DOF block/Subsystem/find the derivative of the quaternion ==
  data: w input; q input; qdot output
function qdot = dquat(w,q)
%#eml
qcrs=[q(4) -q(3) q(2)
      q(3) q(4) -q(1)
      -q(2) q(1) q(4)
      -q(1) -q(2) -q(3)];
qdot=1/2*qcrs*w;

== matlab function Full_system_6DOF/SROA_ rigid_body_dynamics_6DOF/External Damper 6DOF block/Subsystem/quat2DCM ==
  data: q input; DCM output
function DCM = quat2DCM(q)
%#eml
q1=q(1); q2=q(2); q3=q(3); q4=q(4); 

DCM=(q4^2-[q1 q2 q3]*[q1 q2 q3]')*eye(3)+...
    2*[q1 q2 q3]'*[q1 q2 q3]+...
    2*q4*[0 -q3 q2; q3 0 -q1; -q2 q1 0];

== matlab function Full_system_6DOF/image_effect ==
  data: OS_mu input; F_body_images output; OS_xyz input; OS_mu_fc input; fc_xyz input; origin input; tau_body_images output; CoM input; U_images output
function [F_body_images,tau_body_images,U_images]=image_effect(OS_mu,OS_xyz,...
    OS_mu_fc,fc_xyz,origin,CoM)
%#codegen

%F_body_images is the total force on the body due to mobile and frozen
% image effects
%tau_body_images is the total torque on the body due to mobile and frozen
% image effects
%frozen_lists and mobile_lists keeps track of the individual mobile and
% frozen image effects
%OS_mu are the magnetic moment dipoles of the permanent magnets on the OS
%OS_xyz are the magnet positions on the OS
%OS_mu_fc are the field cooled magnetic moment dipoles of the permanent
% magnets on the OS
%fc_xyz are the field cooled positions of the permanent magnets on the OS
%origin is an arbitrary point on the superconductor surface that I have
% chosen to be the center of the superconductor disk surface

%F_body_sum and tau_body_sum is to keep track of the communative effort of
%all frozen and mobile images on magnet i, correlating to row i
F_body_sum=zeros(size(OS_mu,1),3);
tau_body_sum=zeros(size(OS_mu,1),3);
U_fsum=zeros(size(OS_mu,1),1);
U_msum=zeros(size(OS_mu,1),1);
%frozen_lists and mobile_lists goes more in depth than F_body_sum and
%tau_body_sum, storing the individual effect of every frozen and mobile
%image where:
%the first column represents magnet i
%the second column represents magnet j
%third to fifth columns represent force on magnet i due to j's image
%sixth to eighth columns represent torque on magnet i due to j's image
% frozen_lists=zeros(size(OS_mu,1)^2,8,size(origin,1));
% mobile_lists=zeros(size(OS_mu,1)^2,8,size(origin,1));


%% Sum frozen and mobile images across different superconductors and all magnets
for k=1:size(origin,1) %sift through all the superconductors
    %initialize row counter
    row=1;
    for i=1:size(OS_xyz,1) %sift through all the magnets i
        
        mu_mag_i=OS_mu(i,:);
        pos_mag_i=OS_xyz(i,:);
        O=origin(k,:);
        
        for j=1:size(OS_xyz,1) %sift through all the magnets j that generate images
            
            mu_mag_j=OS_mu(j,:);
            pos_mag_j=OS_xyz(j,:);
            mu_mag_fc=OS_mu_fc(j,:);
            pos_fc=fc_xyz(j,:);

            %find the contribution of each field cooled image on all the
            %permanent magnets
            effect='frozen';
            [F,tau,U]=calculate_Ftau(mu_mag_i,mu_mag_j,mu_mag_fc,...
                pos_mag_i,pos_mag_j,pos_fc,O,effect);

            F_body_sum(i,:)=F_body_sum(i,:)+F;
            tau_body_sum(i,:)=tau_body_sum(i,:)+tau+cross(pos_mag_i-CoM',F);
            U_fsum(i)=U_fsum(i)+U;
            %this list is for debugging storing all frozen image effects,
            %first column the magnet, second column the frozen image, 3:5
            %column the force, 6:8 the torque
%             frozen_lists(row,1,k)=i;
%             frozen_lists(row,2,k)=j;
%             frozen_lists(row,3:5,k)=F;
%             frozen_lists(row,6:8,k)=tau;      

            %find the contribution of this magnet's mobile image on
            %the i_th source magnet
            effect='mobile';
            [F,tau,U]=calculate_Ftau(mu_mag_i,mu_mag_j,mu_mag_fc,...
                pos_mag_i,pos_mag_j,pos_fc,O,effect);
            
            F_body_sum(i,:)=F_body_sum(i,:)+F;
            tau_body_sum(i,:)=tau_body_sum(i,:)+tau+cross(pos_mag_i-CoM',F);
            U_msum(i)=U_msum(i)+U;
            %this list is for debugging storing all mobile image effects,
            %first column the magnet, second column the frozen image, 3:5
            %column the force, 6:8 the torque
%             mobile_lists(row,1,k)=i;
%             mobile_lists(row,2,k)=j;
%             mobile_lists(row,3:5,k)=F;
%             mobile_lists(row,6:8,k)=tau;

            row=row+1;
        end
    end
end

%sum columns to get the total force and torque on the body
F_body_images=sum(F_body_sum,1)';
tau_body_images=sum(tau_body_sum,1)';
U_images=[sum(U_fsum) sum(U_msum)];

== matlab function Full_system_6DOF/rigid_body_dynamics_6DOF /External Damper 6DOF Block/Subsystem/Initialize quaternion/yaw,pitch,roll to quat ==
  data: q output; angles input
function q = ang2quat(angles)
%#eml
phi=angles(1);
theta=angles(2);
psi=angles(3);
q1=sin(phi/2)*cos(theta/2)*cos(psi/2)-cos(phi/2)*sin(theta/2)*sin(psi/2);
q2=cos(phi/2)*sin(theta/2)*cos(psi/2)+sin(phi/2)*cos(theta/2)*sin(psi/2);
q3=cos(phi/2)*cos(theta/2)*sin(psi/2)-sin(phi/2)*cos(theta/2)*sin(psi/2);
q4=cos(phi/2)*cos(theta/2)*cos(psi/2)+sin(phi/2)*sin(theta/2)*sin(psi/2);
q=[q1 q2 q3 q4]';

== matlab function Full_system_6DOF/rigid_body_dynamics_6DOF /External Damper 6DOF Block/Subsystem/find the derivative of the quaternion ==
  data: w input; q input; qdot output
function qdot = dquat(w,q)
%#eml
qcrs=[q(4) -q(3) q(2)
      q(3) q(4) -q(1)
      -q(2) q(1) q(4)
      -q(1) -q(2) -q(3)];
qdot=1/2*qcrs*w;

== matlab function Full_system_6DOF/rigid_body_dynamics_6DOF /External Damper 6DOF Block/Subsystem/quat2DCM ==
  data: q input; DCM output
function DCM = quat2DCM(q)
%#eml
q1=q(1); q2=q(2); q3=q(3); q4=q(4); 

DCM=(q4^2-[q1 q2 q3]*[q1 q2 q3]')*eye(3)+...
    2*[q1 q2 q3]'*[q1 q2 q3]+...
    2*q4*[0 -q3 q2; q3 0 -q1; -q2 q1 0];

== matlab function Full_system_6DOF/EM_effect ==
  data: V input; OS_mu input; F_body_EM output; OS_xyz input; EM_magmom input; EM_xyz input; tau_body_EM output; CoM input
function [F_body_EM,tau_body_EM]=EM_effect(V,OS_mu,OS_xyz,EM_magmom,EM_xyz,CoM)
%% Calculate the needed electromagnet voltage with a pseudoinverse
    %initialize a placeholder for the pseudoinverse
    A=zeros(6,length(V));
    
    %sift through all the electromagnets to back out portion of force
    %and torque generated from each individually
    for i=1:length(V) 
        %initialize sum of electromagnet contribution acting on each
        %permanent magnet due to electromagnet i
        dF_tot=zeros(1,3); 
        dtau_tot=zeros(1,3);
        %calculate electromagnet affect on force and torque on body through
        %all the permanent magnets
        for j=1:size(OS_xyz,1) 
            %in this case, the magnetic moment dipole being acted on is the 
            %permanent magnet, following Villani convention
            mu_mag_i=OS_mu(j,:);
            pos_mag_i=OS_xyz(j,:);
            %the magnetic moment dipole acting on magnet i is the
            %electromagnet
            mu_mag_j=EM_magmom(i,:);
            pos_mag_j=EM_xyz(i,:);
            %calculate_dV is a variation of villani. Villani requires mu
            %components and the position vector between them. Within
            %calculate_dV, the electromagnet's magnetic dipole/voltage is
            %substituted for force and torque per unit Volt
            [dF_dV,dtau_dV]=calculate_dV(mu_mag_i,pos_mag_i,mu_mag_j,pos_mag_j);
            %sum over each permanent magnet
            dF_tot=dF_tot+dF_dV;
            dtau_tot=dtau_tot+dtau_dV+cross(dF_tot,pos_mag_i-CoM');
        end
        %fill in the portion of the pseudoinverse needed to calculate
        %electromagnetic contribution
        A(:,i)=[dF_tot';dtau_tot'];
    end
    %voltage calculated for this time step using the pseudoinverse
    y=A*V;
    F_body_EM=y(1:3);
    tau_body_EM=y(4:6);
end
    
function [dF_dV,dtau_dV]=calculate_dV(mu_mag_i,pos_mag_i,mu_mag_j,pos_mag_j)
%this function calculates force and torque per voltage acting on the 
%source magnet from an electromagnet
%mu_mag_i is the magnetic moment dipole of a magnet i
%mu_mag_j is the magnetic moment dipole of the electromagnet
%pos_mag_i is the position of the magnet i
%pos_mag_j is the position of the electromagnet

%the following parameters follow Laura's past experiments
%area enclosed by the electromagnet's current loop
A=0.001829214; %m^2
%number of turns in the electromagnet
T=1060;
%resistance of electromagnet
R=16.8; %Ohmsa
%the permeability of free space, mu_0
mu_0=4*pi*10^-7; %N/A^2

%the following parameters are required by Villani's analytical equations
%for forces and torques on two magnetic dipoles
rho_mji=pos_mag_j-pos_mag_i;
mu_mj_dV=A*T/R*mu_mag_j;
%the voltage is directly proportional to the force and torque applied on
%the magnetic dipole, making the calculation linear and relatively easy

[dF_dV,dtau_dV]=villani(mu_0,mu_mj_dV,mu_mag_i,rho_mji);
%the dF_dV dtau_dV will be evaluated for each electromagnet
%where [F; tau]=[dF_dV;dtau_dV]*[V] 
%V is a 6x1 column vector consisting of V_n for electromagnet n
%F is a 3x1 column vector consisting of forces in the x, y, and z
%tau is a 3x1 column vector consisting of torques in the x, y, and z
%[dF_dV;dtau_dV] is a 6x6 matrix consisting of the contribution of force
%and torque per volt from each electromagnet

end
